simulink model "nestedLoopArchitecture_+_Park"  (R2024b)
settings: Solver=VariableStepAuto  StartTime=0.0  StopTime=10.0  RelTol=1e-3
libraries: fl_lib x9, nesl_utility x6, simulink x4, ee_lib x2, eeGeneralControl x2, slpidlib x2
settings Model: Creator=Erik  LastModifiedBy=ftasc
settings RTWCC: GPUComputeCapability=3.5

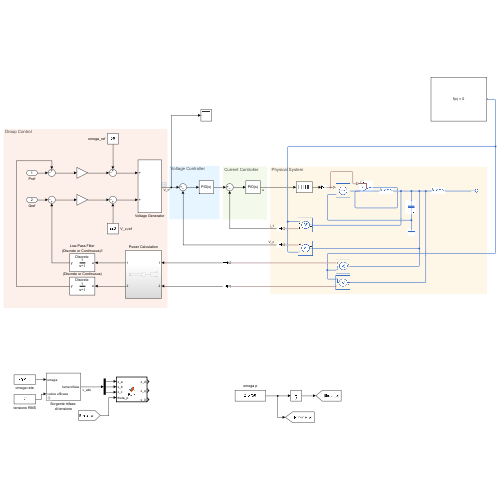
[thumbnail: Simulink's stored preview of the top-level diagram]
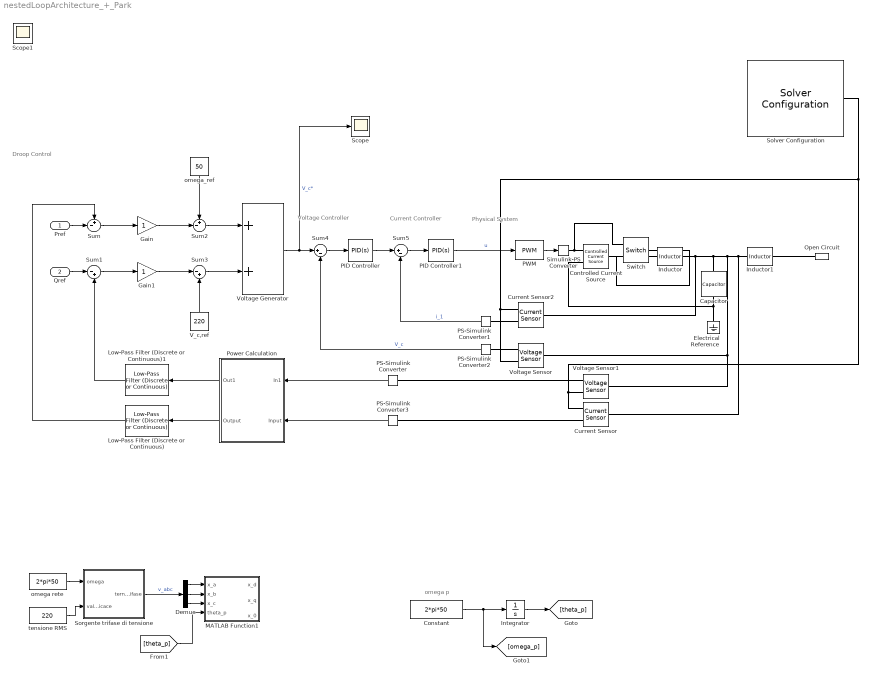
== system nestedLoopArchitecture_+_Park ==
  note: Physical System
  note: Current Controller
  note: Voltage Controller
  note: Droop Control
  note: omega p
  Pref : Inport
  Qref : Inport  Port=2
  Capacitor : fl_lib/Electrical/Electrical Elements/Capacitor  c=1e-6 F  r=1e-6 Ohm  g=0 1/Ohm  i_specify=off  i_priority=None  i=0 A  i_nominal_specify=off  i_nominal_value=1  i_nominal_unit=A  v_specify=off  v_priority=None  v=0 V  v_nominal_specify=off  v_nominal_value=1  v_nominal_unit=V  vc_specify=off  vc_priority=High  vc=0 V  vc_nominal_specify=off  vc_nominal_value=1  vc_nominal_unit=V
  Constant : Constant  Value=2*pi*50
  Controlled Current Source : fl_lib/Electrical/Electrical Sources/Controlled Current Source
  Current Sensor : fl_lib/Electrical/Electrical Sensors/Current Sensor
  Current Sensor2 : fl_lib/Electrical/Electrical Sensors/Current Sensor
  Demux : Demux  Outputs=3
  Electrical Reference : fl_lib/Electrical/Electrical Elements/Electrical Reference
  Gain : Gain
  Gain1 : Gain
  Inductor : ee_lib/Passive/Inductor  l=1e-6 H  enable_L_tol=ee.enum.toleranceApplication.none  L_tol=20  tol_distribution=ee.enum.toleranceDistribution.uniform  nSigma=4  r=0 Ohm  g=1e-9 1/Ohm  enable_operating_limits=ee.enum.enable.no  operating_limit_action=ee.enum.passive.reportOpLim.warn  max_working_current=1 A  power_rating=1 W  fault_action=simscape.enum.assert.action.none  t_fault=1 s  i_L_specify=off  i_L_priority=High  i_L=0 A  i_L_nominal_specify=off  i_L_nominal_value=1  i_L_nominal_unit=A
  Inductor1 : ee_lib/Passive/Inductor  l=1e-6 H  enable_L_tol=ee.enum.toleranceApplication.none  L_tol=20  tol_distribution=ee.enum.toleranceDistribution.uniform  nSigma=4  r=0 Ohm  g=1e-9 1/Ohm  enable_operating_limits=ee.enum.enable.no  operating_limit_action=ee.enum.passive.reportOpLim.warn  max_working_current=1 A  power_rating=1 W  fault_action=simscape.enum.assert.action.none  t_fault=1 s  i_L_specify=off  i_L_priority=High  i_L=0 A  i_L_nominal_specify=off  i_L_nominal_value=1  i_L_nominal_unit=A
  Integrator : Integrator
  Low-Pass Filter (Discrete or Continuous) : eeGeneralControl/Low-Pass Filter (Discrete or Continuous)  K=1  T=1  B=inf  A=-inf  init_option=Inherited from block input  x0=0  Ts=-1
  Low-Pass Filter (Discrete or Continuous)1 : eeGeneralControl/Low-Pass Filter (Discrete or Continuous)  K=1  T=1  B=inf  A=-inf  init_option=Inherited from block input  x0=0  Ts=-1
  MATLAB Function1 : MATLAB Function  TreatAsAtomicUnit=on
  Open Circuit : fl_lib/Electrical/Electrical Elements/Open Circuit  v_specify=off  v_priority=None  v=0 V  v_nominal_specify=off  v_nominal_value=1  v_nominal_unit=V
  PID Controller : slpidlib/PID Controller  Controller=PID  Form=Parallel  TimeDomain=Continuous-time  UseExternalTs=off  SampleTime=-1  IntegratorMethod=Forward Euler  FilterMethod=Forward Euler  ControllerParametersSource=internal  P=1  I=1  UseKiTs=off  D=0  UseExternalDerivativeSource=off  N=100  UseFilter=on  TunerSelectOption=Transfer Function Based (PID Tuner App)  InitialConditionSource=internal  InitialConditionForIntegrator=0  InitialConditionForFilter=0  DifferentiatorICPrevScaledInput=0  ExternalReset=none  TrackingMode=off  Kt=1  LimitOutput=off  SatLimitsSource=internal  UpperSaturationLimit=inf  LowerSaturationLimit=-inf  LinearizeAsGain=on  AntiWindupMode=none  Kb=1  LimitIntegrator=off  UpperIntegratorSaturationLimit=inf  LowerIntegratorSaturationLimit=-inf  POutMin=[]  POutMax=[]  IOutMin=[]  IOutMax=[]  DOutMin=[]  DOutMax=[]  NOutMin=[]  NOutMax=[]  SumOutMin=[]  SumOutMax=[]  SaturationOutMin=[]  SaturationOutMax=[]  PParamMin=[]  PParamMax=[]  IParamMin=[]  IParamMax=[]  DParamMin=[]  DParamMax=[]  NParamMin=[]  NParamMax=[]  KbParamMin=[]  KbParamMax=[]  KtParamMin=[]  KtParamMax=[]  KbOutMin=[]  KbOutMax=[]  KtOutMin=[]  KtOutMax=[]  IntegratorOutMin=[]  IntegratorOutMax=[]  FilterOutMin=[]  FilterOutMax=[]  SumI1OutMin=[]  SumI1OutMax=[]  SumI2OutMin=[]  SumI2OutMax=[]  SumI3OutMin=[]  SumI3OutMax=[]  SumI4OutMin=[]  SumI4OutMax=[]  SumDOutMin=[]  SumDOutMax=[]  DifferentiatorOutMin=[]  DifferentiatorOutMax=[]  FilterDiffOutCoefMin=[]  FilterDiffOutCoefMax=[]  ReciprocalOutMin=[]  ReciprocalOutMax=[]  SumDenOutMin=[]  SumDenOutMax=[]  SumNumOutMin=[]  SumNumOutMax=[]  DivideOutMin=[]  DivideOutMax=[]  UdiffTsProdOutMin=[]  UdiffTsProdOutMax=[]  NTsProdOutMin=[]  NTsProdOutMax=[]  UintegralTsProdOutMin=[]  UintegralTsProdOutMax=[]  UngainTsProdOutMin=[]  UngainTsProdOutMax=[]  ClampingZeroOutDataTypeStr=Inherit: Inherit via back propagation  ClampingZeroOutMin=[]  ClampingZeroOutMax=[]  FilterDenConstantOutDataTypeStr=Inherit: Inherit via back propagation  FilterDenConstantOutMin=[]  FilterDenConstantOutMax=[]  PCopyOutDataTypeStr=Inherit: Inherit via back propagation  PCopyOutMin=[]  PCopyOutMax=[]  NCopyOutDataTypeStr=Inherit: Inherit via back propagation  NCopyOutMin=[]  NCopyOutMax=[]  IntegratorContinuousStateAttributes=''  IntegratorStateMustResolveToSignalObject=off  IntegratorRTWStateStorageClass=Auto  FilterContinuousStateAttributes=''  FilterStateMustResolveToSignalObject=off  FilterRTWStateStorageClass=Auto  ParallelPVariant=InternalParameters  IdealPVariant=Disabled  IVariant=InternalParameters  DVariant=InternalParameters  IntegratorVariant=Continuous  SatVariant=Disabled  AWVariant=Passthrough  PCopyVariant=Disabled  TRVariant=Disabled  FdbkBlocksVariant=Forward  IdealPFdbkVariant=Disabled  SatFdbkVariant=Disabled  DerivativeFilterVariant=ContFilter  NVariant=InternalParameters  NCopyVariant=Disabled  FilterICVariant=InternalICsFilter  IntegratorICVariant=InternalICs  ExternalResetVariant=Disabled  TRSumVariant=Passthrough  SumFdbkVariant=Disabled  SumVariant=Sum_PID  TsampFilterVariant=InternalTs  TsampNgainVariant=Passthrough  TsampIntegralVariant=Disabled_SignalSpec  ExternalSaturationOutDataTypeStr=Inherit: Same as second input  DerivativeSourceVariant=ErrorSignal  PreIntVariant=InternalPreInt
  PID Controller1 : slpidlib/PID Controller  Controller=PID  Form=Parallel  TimeDomain=Continuous-time  UseExternalTs=off  SampleTime=-1  IntegratorMethod=Forward Euler  FilterMethod=Forward Euler  ControllerParametersSource=internal  P=1  I=1  UseKiTs=off  D=0  UseExternalDerivativeSource=off  N=100  UseFilter=on  TunerSelectOption=Transfer Function Based (PID Tuner App)  InitialConditionSource=internal  InitialConditionForIntegrator=0  InitialConditionForFilter=0  DifferentiatorICPrevScaledInput=0  ExternalReset=none  TrackingMode=off  Kt=1  LimitOutput=off  SatLimitsSource=internal  UpperSaturationLimit=inf  LowerSaturationLimit=-inf  LinearizeAsGain=on  AntiWindupMode=none  Kb=1  LimitIntegrator=off  UpperIntegratorSaturationLimit=inf  LowerIntegratorSaturationLimit=-inf  POutMin=[]  POutMax=[]  IOutMin=[]  IOutMax=[]  DOutMin=[]  DOutMax=[]  NOutMin=[]  NOutMax=[]  SumOutMin=[]  SumOutMax=[]  SaturationOutMin=[]  SaturationOutMax=[]  PParamMin=[]  PParamMax=[]  IParamMin=[]  IParamMax=[]  DParamMin=[]  DParamMax=[]  NParamMin=[]  NParamMax=[]  KbParamMin=[]  KbParamMax=[]  KtParamMin=[]  KtParamMax=[]  KbOutMin=[]  KbOutMax=[]  KtOutMin=[]  KtOutMax=[]  IntegratorOutMin=[]  IntegratorOutMax=[]  FilterOutMin=[]  FilterOutMax=[]  SumI1OutMin=[]  SumI1OutMax=[]  SumI2OutMin=[]  SumI2OutMax=[]  SumI3OutMin=[]  SumI3OutMax=[]  SumI4OutMin=[]  SumI4OutMax=[]  SumDOutMin=[]  SumDOutMax=[]  DifferentiatorOutMin=[]  DifferentiatorOutMax=[]  FilterDiffOutCoefMin=[]  FilterDiffOutCoefMax=[]  ReciprocalOutMin=[]  ReciprocalOutMax=[]  SumDenOutMin=[]  SumDenOutMax=[]  SumNumOutMin=[]  SumNumOutMax=[]  DivideOutMin=[]  DivideOutMax=[]  UdiffTsProdOutMin=[]  UdiffTsProdOutMax=[]  NTsProdOutMin=[]  NTsProdOutMax=[]  UintegralTsProdOutMin=[]  UintegralTsProdOutMax=[]  UngainTsProdOutMin=[]  UngainTsProdOutMax=[]  ClampingZeroOutDataTypeStr=Inherit: Inherit via back propagation  ClampingZeroOutMin=[]  ClampingZeroOutMax=[]  FilterDenConstantOutDataTypeStr=Inherit: Inherit via back propagation  FilterDenConstantOutMin=[]  FilterDenConstantOutMax=[]  PCopyOutDataTypeStr=Inherit: Inherit via back propagation  PCopyOutMin=[]  PCopyOutMax=[]  NCopyOutDataTypeStr=Inherit: Inherit via back propagation  NCopyOutMin=[]  NCopyOutMax=[]  IntegratorContinuousStateAttributes=''  IntegratorStateMustResolveToSignalObject=off  IntegratorRTWStateStorageClass=Auto  FilterContinuousStateAttributes=''  FilterStateMustResolveToSignalObject=off  FilterRTWStateStorageClass=Auto  ParallelPVariant=InternalParameters  IdealPVariant=Disabled  IVariant=InternalParameters  DVariant=InternalParameters  IntegratorVariant=Continuous  SatVariant=Disabled  AWVariant=Passthrough  PCopyVariant=Disabled  TRVariant=Disabled  FdbkBlocksVariant=Forward  IdealPFdbkVariant=Disabled  SatFdbkVariant=Disabled  DerivativeFilterVariant=ContFilter  NVariant=InternalParameters  NCopyVariant=Disabled  FilterICVariant=InternalICsFilter  IntegratorICVariant=InternalICs  ExternalResetVariant=Disabled  TRSumVariant=Passthrough  SumFdbkVariant=Disabled  SumVariant=Sum_PID  TsampFilterVariant=InternalTs  TsampNgainVariant=Passthrough  TsampIntegralVariant=Disabled_SignalSpec  ExternalSaturationOutDataTypeStr=Inherit: Same as second input  DerivativeSourceVariant=ErrorSignal  PreIntVariant=InternalPreInt
  PS-Simulink Converter{,1..3} (4 alike) : nesl_utility/PS-Simulink Converter  PhysicalDomain=network_engine_domain  SubClassName=ps_output  LeftPortType=input  RightPortType=output  PseudoPeriodic=off  Frequencies=[]  VectorFormat=inherit  Unit=inherit  AffineConversion=off
  PWM : simulink/Discontinuities/PWM  DisableCoverage=on  Period=1  InitialDelay=0  DisallowZeroDutyCycle=off  RunAtFixedTimeIntervals=off  SampleTime=0.1
  Power Calculation : Subsystem
  Scope : Scope
  Simulink-PS Converter : nesl_utility/Simulink-PS Converter  PhysicalDomain=network_engine_domain  SubClassName=ps_input  LeftPortType=input  RightPortType=output  PseudoPeriodic=off  Frequencies=[]  NoiseDistribution=none  NoiseParameters=[]  Unit=1  AffineConversion=off  FilteringAndDerivatives=provide  SimscapeFilterOrder=1  InputFilterTimeConstant=0.001  UdotUserProvided=0
  Solver Configuration : nesl_utility/Solver Configuration  PhysicalDomain=network_engine_domain  SubClassName=solver  LeftPortType=input  RightPortType=generic  Tones=[]  Harmonics=[]  SimulateNoise=off  Profile=off  UseLocalSampling=off  EnableSwitchedLinearOptims=on  FrequencyDomain=off  UseCCode=off  RelTol=0.001  AbsTol=0.001  MinStep=1e-09  ToWorkspace=off  RevertToSquareIcSolve=off  NumHomotopyIterations=100  PhasorMode=off  PhasorModeNumHarmonics=1  ConsistencySolver=NEWTON_XTOL_AFTER_FTOL  IndexReductionMethod=DerivativeReplacement  DoDC=on  ResidualTolerance=1e-09  ConsistencyTolSource=GLOBAL  ConsistencyAbsTol=0.001  ConsistencyRelTol=0.001  ConsistencyTolFactor=0.001  UseLocalSolver=off  LocalSolverChoice=NE_BACKWARD_EULER_ADVANCER  ResolveIndetEquations=on  FunctionEvalNumThread=1  LocalSolverSampleTime=0.001  DoFixedCost=off  MaxNonlinIter=3  MaxModeIter=2  ComputeImpulses=off  ImpulseIterations=2  LinearAlgebra=auto  LinearAlgebraNumThread=0  EquationFormulation=NE_TIME_EF  DelaysMemoryBudget=1024  AutomaticFiltering=on  FilteringTimeConstant=0.001  PartitionStorageMethod=AS_NEEDED  PartitionMemoryBudget=1024  PartitionMethod=ROBUST  MultibodyUseLocalSolver=off  MultibodyLocalSolverChoice=ODE1  MultibodyLocalSolverSampleTime=0.001
  Sorgente trifase di tensione : Subsystem  mask{onda=Inverter PWM, fsw=10000, DCbus=750}
      mask prompts: onda "Forma d'onda"; fsw "Frequenza di commutazione"; DCbus "Tensione DC bus"
      mask TypeOptions onda: Sinusoidale | Inverter onda quadra | Inverter PWM
      mask Callback onda:
      | onda_block=get_param(gcb,'onda');
      | 
      | if strcmp(onda_block,'Inverter PWM');
      |     set_param(gcb,'MaskVisibilities',{'on';'on';'on'})
      | else
      |     set_param(gcb,'MaskVisibilities',{'on';'off';'off'})
      | end
      mask DialogControl DescGroupVar Prompt: Sorgente trifase di tensione
      mask DialogControl DescTextVar Prompt: Genera una terna trifase con valore efficace e frequenza dati. Si possono selezionare le forme d'onda sinusoidale, onda quadra e PWM
  Sum : Sum  Inputs=+-|
  Sum1 : Sum  Inputs=|-+
  Sum2 : Sum  Inputs=+-|
  Sum3 : Sum  Inputs=|-+
  Sum4 : Sum  Inputs=|+-
  Sum5 : Sum  Inputs=|+-
  Switch : fl_lib/Electrical/Electrical Elements/Switch  R_closed=0.01 Ohm  G_open=1e-8 1/Ohm  Threshold=0.5  i_specify=off  i_priority=None  i=0 A  i_nominal_specify=off  i_nominal_value=1  i_nominal_unit=A  v_specify=off  v_priority=None  v=0 V  v_nominal_specify=off  v_nominal_value=1  v_nominal_unit=V
  V_c,ref : Constant  Value=220
  Voltage Generator : Sum
  Voltage Sensor : fl_lib/Electrical/Electrical Sensors/Voltage Sensor
  Voltage Sensor1 : fl_lib/Electrical/Electrical Sensors/Voltage Sensor
  "omega rete " : Constant  Value=2*pi*50
  omega_ref : Constant  Value=50
  tensione RMS : Constant  Value=220
  Scope1 : Scope
  wires:
  Sum/1 -> Gain/1
  Sum1/1 -> Gain1/1
  Gain1/1 -> Sum3/1
  V_c,ref/1 -> Sum3/2
  Gain/1 -> Sum2/2
  omega_ref/1 -> Sum2/1
  Sum3/1 -> Voltage Generator/2
  Sum2/1 -> Voltage Generator/1
  Voltage Generator/1 -> Scope/1, Sum4/1  "V_c*"
  Sum4/1 -> PID Controller/1
  PID Controller/1 -> Sum5/1
  Power Calculation/1(Out1) -> Low-Pass Filter (Discrete or Continuous)1/1
  Power Calculation/2(Output) -> Low-Pass Filter (Discrete or Continuous)/1
  Low-Pass Filter (Discrete or Continuous)1/1 -> Sum1/2
  Low-Pass Filter (Discrete or Continuous)/1 -> Sum/1
  Pref/1 -> Sum/2
  Qref/1 -> Sum1/1
  PS-Simulink Converter/1 -> Power Calculation/1(In1)
  PWM/1 -> Simulink-PS Converter/1
  Sum5/1 -> PID Controller1/1
  PID Controller1/1 -> PWM/1  "u"
  PS-Simulink Converter1/1 -> Sum5/2  "i_1"
  PS-Simulink Converter2/1 -> Sum4/2  "V_c"
  PS-Simulink Converter3/1 -> Power Calculation/2(Input)
  Constant/1 -> [omega_p], Integrator/1
  Integrator/1 -> [theta_p]
  tensione RMS/1 -> Sorgente trifase di tensione/2(valore efficace)
  "omega rete "/1 -> Sorgente trifase di tensione/1(omega)
  Sorgente trifase di tensione/1(terna trifase) -> Demux/1  "v_abc"
  Demux/2 -> MATLAB Function1/2(x_b)
  Demux/1 -> MATLAB Function1/1(x_a)
  [theta_p] -> MATLAB Function1/4(theta_p)
  Demux/3 -> MATLAB Function1/3(x_c)
  connections:
  Electrical Reference/LConn1 -- Controlled Current Source/RConn2 -- Capacitor/RConn1
  Inductor/RConn1 -- Current Sensor2/LConn1 -- Voltage Sensor/LConn1 -- Voltage Sensor1/LConn1 -- Current Sensor/LConn1 -- Inductor1/LConn1 -- Capacitor/LConn1
  Controlled Current Source/RConn1 -- Switch/RConn1 -- Simulink-PS Converter/RConn1
  Current Sensor/RConn1 -- PS-Simulink Converter3/LConn1
  Open Circuit/LConn1 -- Inductor1/RConn1
  Current Sensor2/RConn1 -- PS-Simulink Converter1/LConn1
  Voltage Sensor1/RConn1 -- PS-Simulink Converter/LConn1
  Voltage Sensor/RConn1 -- PS-Simulink Converter2/LConn1
  Controlled Current Source/LConn1 -- Switch/RConn2
  Switch/LConn1 -- Inductor/LConn1
  Voltage Sensor1/RConn2 -- Voltage Sensor/RConn2 -- Current Sensor2/RConn2 -- Solver Configuration/RConn1 -- Current Sensor/RConn2

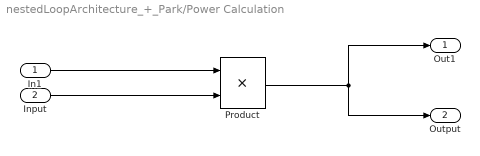
== system nestedLoopArchitecture_+_Park/Power Calculation ==
  In1 : Inport
  Input : Inport  Port=2
  Product : Product
  Out1 : Outport
  Output : Outport  Port=2
  wires:
  In1/1 -> Product/1
  Input/1 -> Product/2
  Product/1 -> Output/1, Out1/1

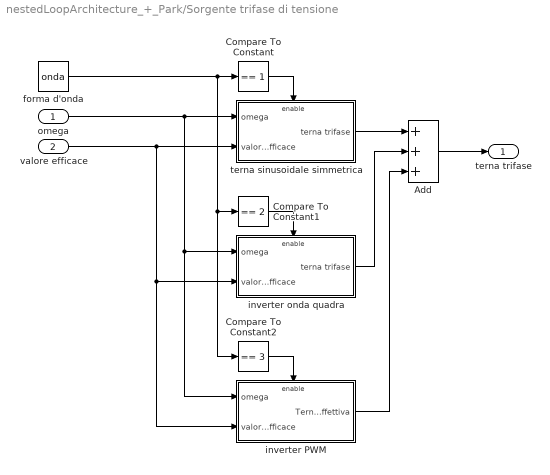
== system nestedLoopArchitecture_+_Park/Sorgente trifase di tensione ==
  omega : Inport
  valore efficace : Inport  Port=2
  Add : Sum  Inputs=3
  Compare To Constant : simulink/Logic and Bit Operations/Compare To Constant  relop===  const=1  OutDataTypeStr=boolean
  Compare To Constant1 : simulink/Logic and Bit Operations/Compare To Constant  relop===  const=2  OutDataTypeStr=boolean
  Compare To Constant2 : simulink/Logic and Bit Operations/Compare To Constant  relop===  const=3  OutDataTypeStr=boolean
  forma d'onda : Constant  Value=onda
  inverter PWM : Subsystem  TreatAsAtomicUnit=on  mask{Vdc=DCbus, f_sw=fsw}
      mask prompts: Vdc "Tensione del dc bus"; f_sw "Frequenza di switching"
  inverter onda quadra : Subsystem  TreatAsAtomicUnit=on
  terna sinusoidale simmetrica : Subsystem  TreatAsAtomicUnit=on
  terna trifase : Outport  VectorParamsAs1DForOutWhenUnconnected=off
  wires:
  valore efficace/1 -> terna sinusoidale simmetrica/2(valore efficace), inverter onda quadra/2(valore efficace), inverter PWM/2(valore efficace)
  omega/1 -> terna sinusoidale simmetrica/1(omega), inverter onda quadra/1(omega), inverter PWM/1(omega)
  Compare To Constant/1 -> terna sinusoidale simmetrica/Enable
  Compare To Constant1/1 -> inverter onda quadra/Enable
  Compare To Constant2/1 -> inverter PWM/Enable
  forma d'onda/1 -> Compare To Constant2/1, Compare To Constant1/1, Compare To Constant/1
  terna sinusoidale simmetrica/1(terna trifase) -> Add/1
  inverter onda quadra/1(terna trifase) -> Add/2
  inverter PWM/1(Terna effettiva) -> Add/3
  Add/1 -> terna trifase/1

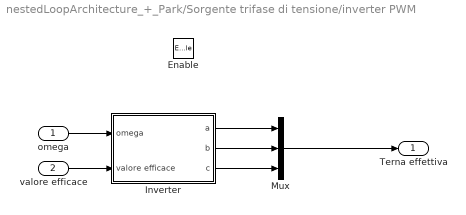
== system nestedLoopArchitecture_+_Park/Sorgente trifase di tensione/inverter PWM ==
  omega : Inport
  valore efficace : Inport  Port=2
  Enable : EnablePort
  Inverter : Subsystem  mask{Vdc=Vdc, f_sw=f_sw}
      mask prompts: Vdc "Tensione nominale del dc bus"; f_sw "Frequenza di switching"
  Mux : Mux  Inputs=3
  Terna effettiva : Outport  VectorParamsAs1DForOutWhenUnconnected=off
  wires:
  valore efficace/1 -> Inverter/2(valore efficace)
  omega/1 -> Inverter/1(omega)
  Mux/1 -> Terna effettiva/1
  Inverter/3(c) -> Mux/3
  Inverter/1(a) -> Mux/1
  Inverter/2(b) -> Mux/2

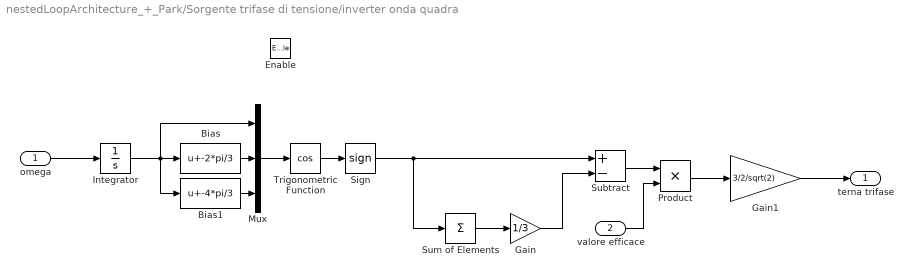
== system nestedLoopArchitecture_+_Park/Sorgente trifase di tensione/inverter onda quadra ==
  omega : Inport
  valore efficace : Inport  Port=2
  Enable : EnablePort
  Bias : Bias  Bias=-2*pi/3  SaturateOnIntegerOverflow=off
  Bias1 : Bias  Bias=-4*pi/3  SaturateOnIntegerOverflow=off
  Gain : Gain  Gain=1/3
  Gain1 : Gain  Gain=3/2/sqrt(2)
  Integrator : Integrator
  Mux : Mux  Inputs=3
  Product : Product
  Sign : Signum
  Subtract : Sum  Inputs=+-
  Sum of Elements : Sum  Inputs=+
  Trigonometric Function : Trigonometry  Operator=cos
  terna trifase : Outport  VectorParamsAs1DForOutWhenUnconnected=off
  wires:
  Product/1 -> Gain1/1
  Gain1/1 -> terna trifase/1
  valore efficace/1 -> Product/2
  Subtract/1 -> Product/1
  Integrator/1 -> Mux/1, Bias1/1, Bias/1
  Sum of Elements/1 -> Gain/1
  Sign/1 -> Subtract/1, Sum of Elements/1
  Bias1/1 -> Mux/3
  Bias/1 -> Mux/2
  omega/1 -> Integrator/1
  Gain/1 -> Subtract/2
  Trigonometric Function/1 -> Sign/1
  Mux/1 -> Trigonometric Function/1

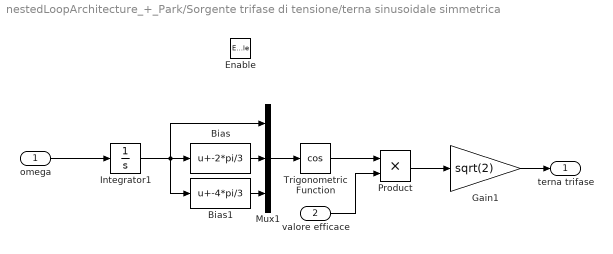
== system nestedLoopArchitecture_+_Park/Sorgente trifase di tensione/terna sinusoidale simmetrica ==
  omega : Inport
  valore efficace : Inport  Port=2
  Enable : EnablePort
  Bias : Bias  Bias=-2*pi/3  SaturateOnIntegerOverflow=off
  Bias1 : Bias  Bias=-4*pi/3  SaturateOnIntegerOverflow=off
  Gain1 : Gain  Gain=sqrt(2)
  Integrator1 : Integrator
  Mux1 : Mux  Inputs=3
  Product : Product
  Trigonometric Function : Trigonometry  Operator=cos
  terna trifase : Outport  VectorParamsAs1DForOutWhenUnconnected=off
  wires:
  valore efficace/1 -> Product/2
  Trigonometric Function/1 -> Product/1
  Bias/1 -> Mux1/2
  omega/1 -> Integrator1/1
  Product/1 -> Gain1/1
  Gain1/1 -> terna trifase/1
  Integrator1/1 -> Mux1/1, Bias1/1, Bias/1
  Bias1/1 -> Mux1/3
  Mux1/1 -> Trigonometric Function/1

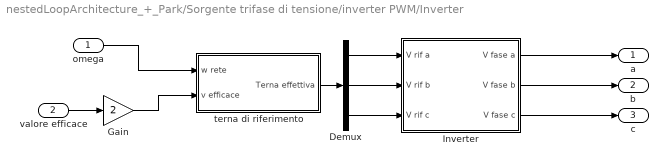
== system nestedLoopArchitecture_+_Park/Sorgente trifase di tensione/inverter PWM/Inverter ==
  omega : Inport
  valore efficace : Inport  Port=2
  Demux : Demux  Outputs=3
  Gain : Gain  Gain=2
  Inverter : Subsystem  mask{Vdc=Vdc, f_sw=f_sw}
      mask prompts: Vdc "tensione nominale del dc-bus"; f_sw "frequenza di switching della portante"
  terna di riferimento : Subsystem
  a : Outport  VectorParamsAs1DForOutWhenUnconnected=off
  b : Outport  Port=2  VectorParamsAs1DForOutWhenUnconnected=off
  c : Outport  Port=3  VectorParamsAs1DForOutWhenUnconnected=off
  wires:
  Inverter/1(V fase a) -> a/1
  Inverter/3(V fase c) -> c/1
  Inverter/2(V fase b) -> b/1
  terna di riferimento/1(Terna effettiva) -> Demux/1
  Demux/2 -> Inverter/2(V rif b)
  Demux/3 -> Inverter/3(V rif c)
  Demux/1 -> Inverter/1(V rif a)
  omega/1 -> terna di riferimento/1(w rete)
  valore efficace/1 -> Gain/1
  Gain/1 -> terna di riferimento/2(v efficace)

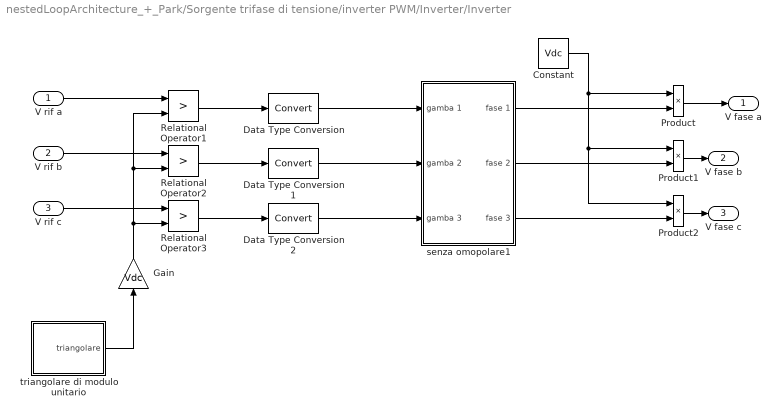
== system nestedLoopArchitecture_+_Park/Sorgente trifase di tensione/inverter PWM/Inverter/Inverter ==
  V rif a : Inport
  V rif b : Inport  Port=2
  V rif c : Inport  Port=3
  Constant : Constant  Value=Vdc
  Data Type Conversion : DataTypeConversion  SaturateOnIntegerOverflow=off  RndMeth=Floor
  Data Type Conversion1 : DataTypeConversion  SaturateOnIntegerOverflow=off  RndMeth=Floor
  Data Type Conversion2 : DataTypeConversion  SaturateOnIntegerOverflow=off  RndMeth=Floor
  Gain : Gain  Gain=Vdc  SaturateOnIntegerOverflow=on  OutDataTypeStr=Inherit: Same as input  ParamDataTypeStr=Inherit: Same as input
  Product : Product  InputSameDT=on  RndMeth=Zero  SaturateOnIntegerOverflow=on  OutDataTypeStr=Inherit: Same as first input
  Product1 : Product  InputSameDT=on  RndMeth=Zero  SaturateOnIntegerOverflow=on  OutDataTypeStr=Inherit: Same as first input
  Product2 : Product  InputSameDT=on  RndMeth=Zero  SaturateOnIntegerOverflow=on  OutDataTypeStr=Inherit: Same as first input
  Relational Operator1 : RelationalOperator  Operator=>
  Relational Operator2 : RelationalOperator  Operator=>
  Relational Operator3 : RelationalOperator  Operator=>
  senza omopolare1 : Subsystem
  triangolare di modulo unitario : Subsystem
  V fase a : Outport  VectorParamsAs1DForOutWhenUnconnected=off
  V fase b : Outport  Port=2  VectorParamsAs1DForOutWhenUnconnected=off
  V fase c : Outport  Port=3  VectorParamsAs1DForOutWhenUnconnected=off
  wires:
  Constant/1 -> Product/1, Product1/1, Product2/1
  V rif a/1 -> Relational Operator1/1
  Product/1 -> V fase a/1
  V rif b/1 -> Relational Operator2/1
  Product1/1 -> V fase b/1
  V rif c/1 -> Relational Operator3/1
  Product2/1 -> V fase c/1
  Gain/1 -> Relational Operator1/2, Relational Operator2/2, Relational Operator3/2
  triangolare di modulo unitario/1(triangolare) -> Gain/1
  Relational Operator1/1 -> Data Type Conversion/1
  Relational Operator2/1 -> Data Type Conversion1/1
  Relational Operator3/1 -> Data Type Conversion2/1
  senza omopolare1/1(fase 1) -> Product/2
  senza omopolare1/2(fase 2) -> Product1/2
  senza omopolare1/3(fase 3) -> Product2/2
  Data Type Conversion/1 -> senza omopolare1/1(gamba 1)
  Data Type Conversion1/1 -> senza omopolare1/2(gamba 2)
  Data Type Conversion2/1 -> senza omopolare1/3(gamba 3)

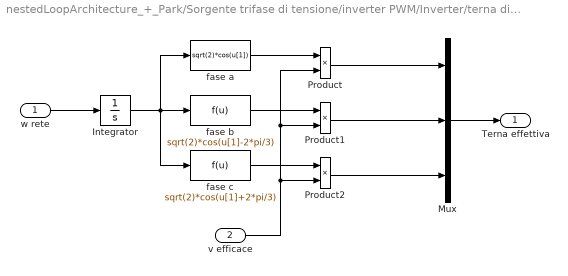
== system nestedLoopArchitecture_+_Park/Sorgente trifase di tensione/inverter PWM/Inverter/terna di riferimento ==
  w rete : Inport
  v efficace : Inport  Port=2
  Integrator : Integrator
  Mux : Mux  Inputs=3
  Product : Product  InputSameDT=on  RndMeth=Zero  SaturateOnIntegerOverflow=on  OutDataTypeStr=Inherit: Same as first input
  Product1 : Product  InputSameDT=on  RndMeth=Zero  SaturateOnIntegerOverflow=on  OutDataTypeStr=Inherit: Same as first input
  Product2 : Product  InputSameDT=on  RndMeth=Zero  SaturateOnIntegerOverflow=on  OutDataTypeStr=Inherit: Same as first input
  "fase a " : Fcn  Expr=sqrt(2)*cos(u[1])
  "fase b " : Fcn  Expr=sqrt(2)*cos(u[1]-2*pi/3)
  "fase c " : Fcn  Expr=sqrt(2)*cos(u[1]+2*pi/3)
  Terna effettiva : Outport  VectorParamsAs1DForOutWhenUnconnected=off
  wires:
  Integrator/1 -> "fase b "/1, "fase a "/1, "fase c "/1
  w rete/1 -> Integrator/1
  "fase a "/1 -> Product/1
  "fase c "/1 -> Product2/1
  "fase b "/1 -> Product1/1
  Product/1 -> Mux/1
  Product1/1 -> Mux/2
  Product2/1 -> Mux/3
  v efficace/1 -> Product/2, Product1/2, Product2/2
  Mux/1 -> Terna effettiva/1

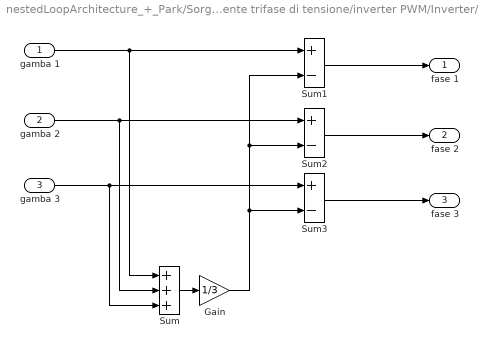
== system nestedLoopArchitecture_+_Park/Sorgente trifase di tensione/inverter PWM/Inverter/Inverter/senza omopolare1 ==
  gamba 1 : Inport
  gamba 2 : Inport  Port=2
  gamba 3 : Inport  Port=3
  Gain : Gain  Gain=1/3  SaturateOnIntegerOverflow=on  OutDataTypeStr=Inherit: Same as input  ParamDataTypeStr=Inherit: Same as input
  Sum : Sum  Inputs=+++  InputSameDT=on  SaturateOnIntegerOverflow=on  OutDataTypeStr=Inherit: Same as first input
  Sum1 : Sum  Inputs=+-  InputSameDT=on  SaturateOnIntegerOverflow=on  OutDataTypeStr=Inherit: Same as first input
  Sum2 : Sum  Inputs=+-  InputSameDT=on  SaturateOnIntegerOverflow=on  OutDataTypeStr=Inherit: Same as first input
  Sum3 : Sum  Inputs=+-  InputSameDT=on  SaturateOnIntegerOverflow=on  OutDataTypeStr=Inherit: Same as first input
  fase 1 : Outport  VectorParamsAs1DForOutWhenUnconnected=off
  fase 2 : Outport  Port=2  VectorParamsAs1DForOutWhenUnconnected=off
  fase 3 : Outport  Port=3  VectorParamsAs1DForOutWhenUnconnected=off
  wires:
  Sum/1 -> Gain/1
  Sum1/1 -> fase 1/1
  gamba 1/1 -> Sum1/1, Sum/1
  Sum2/1 -> fase 2/1
  gamba 2/1 -> Sum2/1, Sum/2
  Sum3/1 -> fase 3/1
  gamba 3/1 -> Sum3/1, Sum/3
  Gain/1 -> Sum1/2, Sum2/2, Sum3/2

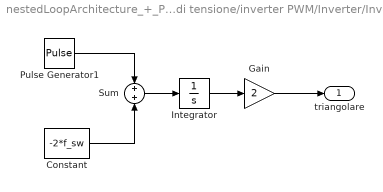
== system nestedLoopArchitecture_+_Park/Sorgente trifase di tensione/inverter PWM/Inverter/Inverter/triangolare di modulo unitario ==
  Constant : Constant  Value=-2*f_sw
  Gain : Gain  Gain=2  SaturateOnIntegerOverflow=on  OutDataTypeStr=Inherit: Same as input  ParamDataTypeStr=Inherit: Same as input
  Integrator : Integrator  InitialCondition=-.5
  Pulse Generator1 : DiscretePulseGenerator  PulseType=Time based  Amplitude=4*f_sw  Period=1/f_sw  PulseWidth=50
  Sum : Sum  InputSameDT=on  SaturateOnIntegerOverflow=on  OutDataTypeStr=Inherit: Same as first input
  triangolare : Outport  VectorParamsAs1DForOutWhenUnconnected=off
  wires:
  Pulse Generator1/1 -> Sum/1
  Sum/1 -> Integrator/1
  Constant/1 -> Sum/2
  Integrator/1 -> Gain/1
  Gain/1 -> triangolare/1

== matlab function nestedLoopArchitecture_+_Park/MATLAB Function1 ==
  data: x_a input; x_d output; x_b input; x_c input; theta_p input; x_q output; x_0 output
function [ x_d , x_q , x_0 ] = Park( x_a , x_b , x_c, theta_p)
% Trasformazione di Park
%   x_a,x_b,x_c    sono le grandezze di fase (fase a, fase b, fase c)
%   x_d,x_q,x_0    sono le componenti disposte su asse diretto, asse in
%                  quadratura, e omopolare rispettivamente
%   theta_p        è l'angolo del sistema di riferimento di Park

Tp = sqrt(2/3) *[ cos(theta_p ) cos(theta_p-2*pi/3)     cos(theta_p-4*pi/3)
                  -sin(theta_p)  -sin(theta_p-2*pi/3)   -sin(theta_p-4*pi/3)
                  1/sqrt(2)           1/sqrt(2)                 1/sqrt(2) ];

x_dq0 = Tp *   [  x_a ;
                  x_b ;
                  x_c ];

x_d = x_dq0 (1);    x_q =x_dq0(2);    x_0 =x_dq0(3);
